simulink model "FSK"  (Simulink 8.9)
settings: Solver=ode45  StartTime=0.0  StopTime=100  RelTol=1e-3  EnableMultiTasking=on
libraries: dsparch4 x2, commrandsrc2 x1
settings Model: Creator=Abhishek  LastModifiedBy=JBlanco
settings DataIOCC: SignalLoggingSaveFormat=Dataset
settings DebuggingCC: SolverPrmCheckMsg=warning  FcnCallInpInsideContextMsg=error
settings GRTTargetCC: CombineOutputUpdateFcns=on  GRTInterface=off

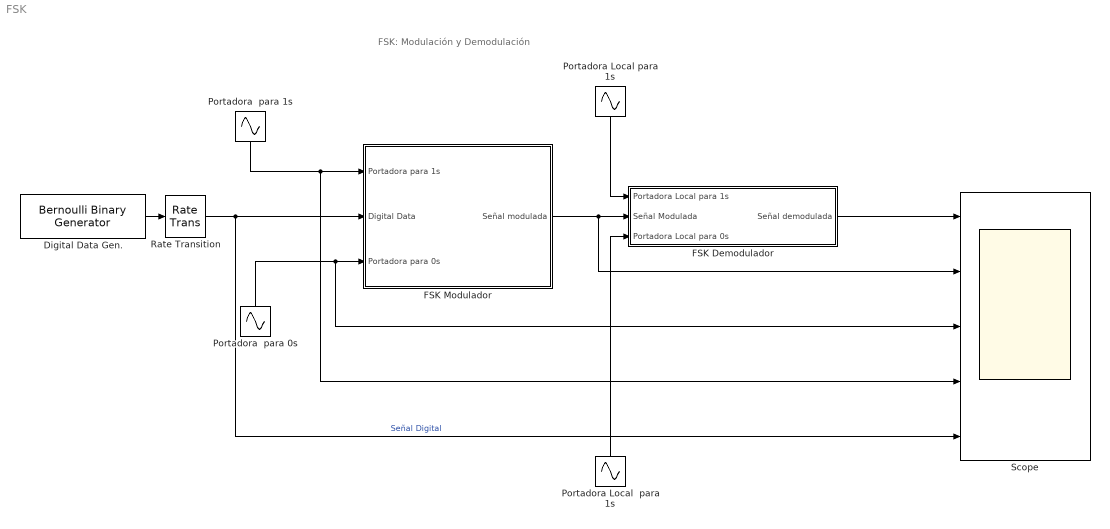
== system FSK ==
  note: FSK: Modulación y Demodulación
  Digital Data Gen. : commrandsrc2/Bernoulli Binary Generator  P=0.5  seed=61  Ts=5  frameBased=off  sampPerFrame=1  orient=off  outDataType=double  mask(Bernoulli Binary Generator){}
      mask Display:
      | % This is a new mask on top of the base mask.
      | % Use "View base mask" link below to see the base mask.
      | disp('Digital Msg Signal')
  FSK Demodulador : Subsystem
  FSK Modulador : Subsystem
  Portadora  para 0s : Sin  Amplitude=5  Frequency=20*2*pi  Samples=50  SampleTime=1/2000
  Portadora  para 1s : Sin  Amplitude=5  Frequency=10*2*pi  Samples=20  SampleTime=1/2000
  Portadora Local para 1s : Sin  Amplitude=5  Frequency=10*2*pi  Samples=20  SampleTime=1/2000
  Portadora Local  para 1s : Sin  Amplitude=5  Frequency=20*2*pi  Samples=50  SampleTime=1/2000
  Rate Transition : RateTransition  OutPortSampleTime=1/2000
  Scope : Scope  NumInputPorts=5
  wires:
  Digital Data Gen./1 -> Rate Transition/1
  FSK Modulador/1(Señal modulada) -> Scope/2, FSK Demodulador/2("Señal Modulada ")
  Portadora  para 1s/1 -> Scope/4, FSK Modulador/1(Portadora para 1s)
  Portadora  para 0s/1 -> Scope/3, FSK Modulador/3(Portadora para 0s)
  FSK Demodulador/1(Señal demodulada) -> Scope/1
  Rate Transition/1 -> Scope/5, FSK Modulador/2(Digital Data)  "Señal Digital"
  Portadora Local para 1s/1 -> FSK Demodulador/1(Portadora Local para 1s)
  Portadora Local  para 1s/1 -> FSK Demodulador/3(Portadora Local para 0s)

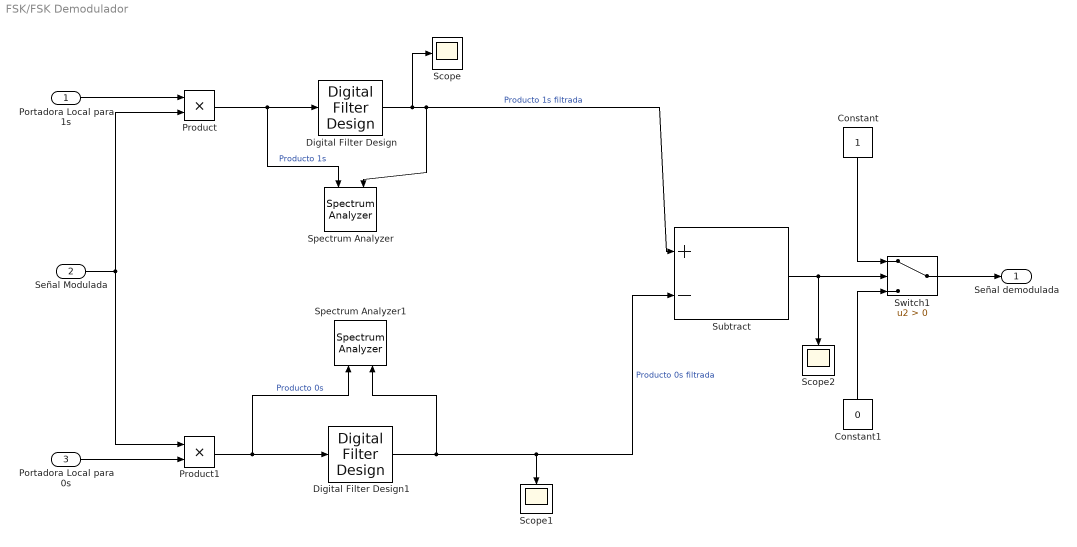
== system FSK/FSK Demodulador ==
  Portadora Local para 1s : Inport
  "Señal Modulada " : Inport  Port=2
  Portadora Local para 0s : Inport  Port=3
  Constant : Constant
  Constant1 : Constant  Value=0
  Digital Filter Design : dsparch4/Digital Filter Design  mwdsp_browser_bugfix_var=off
  Digital Filter Design1 : dsparch4/Digital Filter Design  mwdsp_browser_bugfix_var=off
  Product : Product
  Product1 : Product
  Scope : Scope
  Scope1 : Scope
  Scope2 : Scope
  Spectrum Analyzer : SpectrumAnalyzer  NumInputPorts=2
  Spectrum Analyzer1 : SpectrumAnalyzer  NumInputPorts=2
  Subtract : Sum  Inputs=+-
  Switch1 : Switch  Criteria=u2 > Threshold
  Señal demodulada : Outport
  wires:
  "Señal Modulada "/1 -> Product/2, Product1/1
  Portadora Local para 1s/1 -> Product/1
  Portadora Local para 0s/1 -> Product1/2
  Subtract/1 -> Scope2/1, Switch1/2
  Constant/1 -> Switch1/1
  Constant1/1 -> Switch1/3
  Switch1/1 -> Señal demodulada/1
  Product/1 -> Spectrum Analyzer/1, Digital Filter Design/1  "Producto 1s"
  Digital Filter Design/1 -> Scope/1, Spectrum Analyzer/2, Subtract/1  "Producto 1s filtrada"
  Digital Filter Design1/1 -> Spectrum Analyzer1/2, Subtract/2, Scope1/1  "Producto 0s filtrada"
  Product1/1 -> Digital Filter Design1/1, Spectrum Analyzer1/1  "Producto 0s"

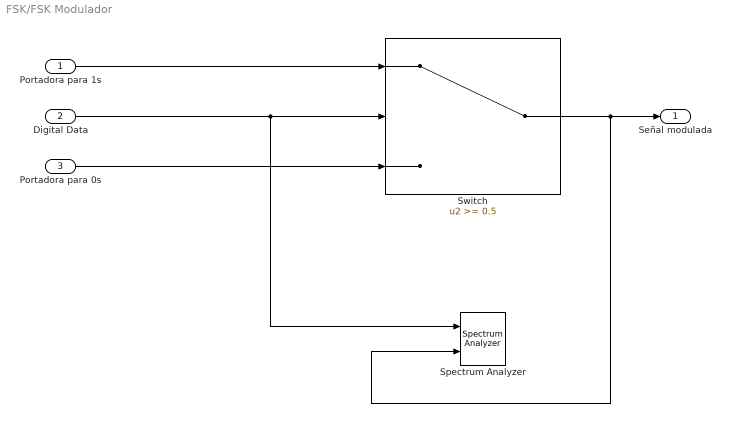
== system FSK/FSK Modulador ==
  Portadora para 1s : Inport
  Digital Data : Inport  Port=2
  Portadora para 0s : Inport  Port=3
  Spectrum Analyzer : SpectrumAnalyzer  NumInputPorts=2
  Switch : Switch  Threshold=0.5
  Señal modulada : Outport
  wires:
  Digital Data/1 -> Spectrum Analyzer/1, Switch/2
  Portadora para 1s/1 -> Switch/1
  Portadora para 0s/1 -> Switch/3
  Switch/1 -> Spectrum Analyzer/2, Señal modulada/1
